simulink model "testbench_fwd_steering"  (R2016a)
settings: Solver=FixedStepAuto  StartTime=0.0  StopTime=inf  RelTol=1e-3
libraries: legoev3lib x5
settings Model: SimulationMode=external  ExtModeTrigDuration=2  Creator=Shobhit  LastModifiedBy=Shobhit
settings SolverCC: PositivePriorityOrder=on
settings OptimizationCC: OptimizeModelRefInitCode=on  LifeSpan=1  MaxStackSize=64
settings HardwareCC: ProdBitPerPointer=32  ProdLargestAtomicInteger=Long  ProdWordSize=32  ProdHWDeviceType=ARM Compatible->ARM 9  UseEmbeddedCoderFeatures=off  UseSimulinkCoderFeatures=off
settings RTWCC: SystemTargetFile=ert.tlc  HardwareBoard=LEGO MINDSTORMS EV3  TemplateMakefile=ert_default_tmf  GenerateReport=on  Toolchain=Sourcery G++ Lite v2009q3  IncludeHyperlinkInReport=on  LaunchReport=on  GenerateTraceInfo=on  GenerateTraceReport=on  GenerateTraceReportSl=on  GenerateTraceReportSf=on  GenerateTraceReportEml=on
settings CodeAppCC: ForceParamTrailComments=on  IgnoreCustomStorageClasses=off  OperatorAnnotations=on  SimulinkDataObjDesc=on  SFDataObjDesc=on  MATLABFcnDesc=on  InsertBlockDesc=on  MATLABSourceComments=on
settings ERTTargetCC: SupportContinuousTime=on  SupportNonInlinedSFcns=on  SupportVariableSizeSignals=on

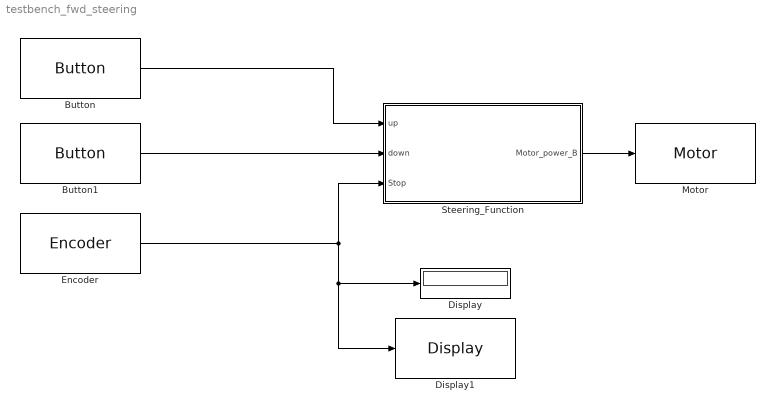
== system testbench_fwd_steering ==
  " Steering_Function" : MATLAB Function  TreatAsAtomicUnit=on
  Button : legoev3lib/Button  buttonType=Up  sampleTime=0.1
  Button1 : legoev3lib/Button  buttonType=Down  sampleTime=0.1
  Display : Display
      settings: Format=decimal (Stored Integer)
  Display1 : legoev3lib/Display  slcdStr=enc A  slcdLine=1  slcdFormat=Decimal
  Encoder : legoev3lib/Encoder  portNumber=B  opMode=No reset  sampleTime=0.1
  Motor : legoev3lib/Motor  sportNumber=B  sstopAction=Brake
  wires:
  " Steering_Function"/1(Motor_power_B) -> Motor/1
  Encoder/1 -> Display1/1, Display/1, " Steering_Function"/3(Stop)
  Button/1 -> " Steering_Function"/1(up)
  Button1/1 -> " Steering_Function"/2(down)

== matlab function testbench_fwd_steering/ Steering_Function ==
  data: up input; down input; Motor_power_B output; Stop input
function Motor_power_B=fcn(up,down,Stop)
%#codegen
if(up==1)&&(Stop<=225)
    Motor_power_B=70;
elseif(down==1)&&(Stop>=-225)
    Motor_power_B=-70;
else
   Motor_power_B=0;
end
end
